simulink model "fuel_cell_vi_model"  (R2025a)
settings: Solver=VariableStepAuto  StartTime=0.0  StopTime=sim_time_duration  RelTol=1e-3
undefined symbols (not defined in the file): A_conc, E_ocv, I_end_sim, I_limit, I_start_sim, N_cells, R_ohmic, sim_time_duration, V_act
libraries: simulink x1
settings Model: Creator=Maintenant prêt  LastModifiedBy=Maintenant prêt

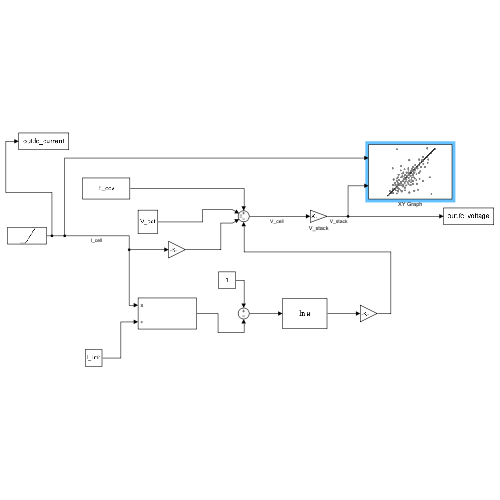
[thumbnail: Simulink's stored preview of the top-level diagram]
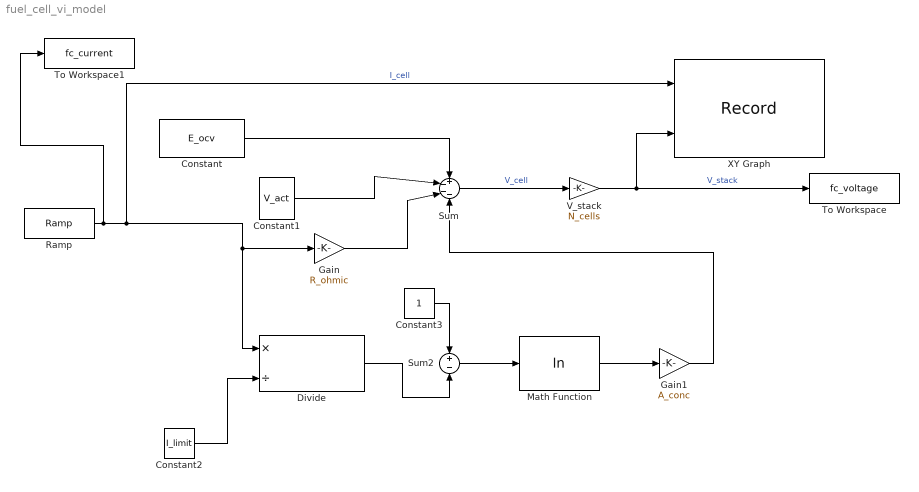
== system fuel_cell_vi_model ==
  Constant : Constant  Value=E_ocv
  Constant1 : Constant  Value=V_act
  Constant2 : Constant  Value=I_limit  VectorParams1D=off
  Constant3 : Constant
  Divide : Product  Inputs=*/  CollapseMode=Specified dimension  InputSameDT=on
  Gain : Gain  Gain=R_ohmic
  Gain1 : Gain  Gain=A_conc
  Math Function : Math  Operator=log  OutputSignalType=real
  Ramp : simulink/Sources/Ramp  slope=(I_end_sim - I_start_sim) / sim_time_duration  start=0  InitialOutput=I_start_sim
  Sum : Sum  Inputs=+---
  Sum2 : Sum  Inputs=+-
  To Workspace : ToWorkspace  VariableName=fc_voltage  SampleTime=-1
  To Workspace1 : ToWorkspace  VariableName=fc_current  SampleTime=-1
  V_stack : Gain  Gain=N_cells
  XY Graph : Record  NumPorts=2.0  FileSettingsInternal="{\"entries\":[{\"content\":{\"excelSettings\":{\"content\":{},\"type\":\"Streamout.ExcelSettings\"},\"parquetSettings\":{\"content\":{},\"type\":\"Streamout.ParquetSettings\"}},\"type\":\"Streamout.FileSettingStorage\",\"uuid\":\"\"}],\"packageUris\":[\"http:\\/\\/schema.mathworks.com\\/mf0\\/streamout_blocks\\/R2020a\"],\"version\":\"1.0\"}"  FrameSettings=[0, 0]  Layout=[1 1]  SignalsInternal="{\"entries\":[{\"content\":{\"signals\":[{\"content\":{\"blockPath\":[],\"dimensions\":[1],\"domain\":\"\",\"lineColor\":\"#a2142f\",\"port\":1,\"sid\":[\"\"],\"signalID\":1,\"signalName\":\"I_cell\"},\"type\":\"RecordBlkView.Signal\",\"uuid\":\"\"},{\"content\":{\"blockPath\":[],\"dimensions\":[1,1],\"domain\":\"\",\"hasChildren\":true,\"isComplex\":true,\"lineColor\":\"#b746ff\",\"lineWidth\":2,\"port\":2,\"sid\":[\"\"],\"signalID\":2,\"signalName\":\"V_stack\"},\"type\":\"RecordBlkView.Signal\",\"uuid\":\"\"},{\"content\":{\"blockPath\":[],\"dimensions\":[1,1],\"domain\":\"\",\"isComplex\":true,\"lineColor\":\"#139fff\",\"parentID\":2,\"port\":2,\"sid\":[\"\"],\"signalID\":3,\"signalName\":\"V_stack\"},\"type\":\"RecordBlkView.Signal\",\"uuid\":\"\"},{\"content\":{\"blockPath\":[],\"dimensions\":[1,1],\"domain\":\"\",\"imagPart\":true,\"isComplex\":true,\"lineColor\":\"#ff13a6\",\"lineWidth\":2,\"parentID\":2,\"port\":2,\"sid\":[\"\"],\"signalID\":4,\"signalName\":\"V_stack\"},\"type\":\"RecordBlkView.Signal\",\"uuid\":\"\"}]},\"type\":\"RecordBlkView.InputSignals\",\"uuid\":\"\"}],\"packageUris\":[\"http:\\/\\/schema.mathworks.com\\/mf0\\/streamout_blocks\\/R2020a\"],\"version\":\"1.0\"}"  VisualizationBindings="{\"xyplotplugin\":{\"info\":[{\"series\":[],\"subplotID\":1}]}}"  CompatibilityTag=XY
  wires:
  Constant/1 -> Sum/1
  Constant1/1 -> Sum/2
  Ramp/1 -> To Workspace1/1, XY Graph/1, Gain/1, Divide/1  "I_cell"
  Gain/1 -> Sum/3
  Constant3/1 -> Sum2/1
  Divide/1 -> Sum2/2
  Sum2/1 -> Math Function/1
  Math Function/1 -> Gain1/1
  Gain1/1 -> Sum/4
  Sum/1 -> V_stack/1  "V_cell"
  V_stack/1 -> To Workspace/1, XY Graph/2  "V_stack"
  Constant2/1 -> Divide/2
